simulink model "quatercar_suspension"  (R2022b)
settings: Solver=VariableStepAuto  StartTime=0.0  StopTime=10.0  RelTol=1e-3
undefined symbols (not defined in the file or in its folder): c, k, m
settings Model: Creator=admin  LastModifiedBy=admin
settings SolverCC: AlgebraicLoopSolver=TrustRegion
settings DebuggingCC: UnconnectedInputMsg=warning  UnconnectedOutputMsg=warning  UnconnectedLineMsg=warning  SFMachineParentedDataDiag=warning
settings ModelReferenceCC: EnableRefExpFcnMdlSchedulingChecks=on
settings RTWCC: DLArmComputeVersion=19.05

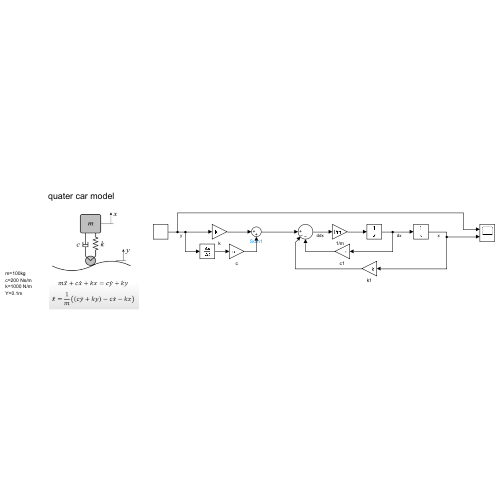
[thumbnail: Simulink's stored preview of the top-level diagram]
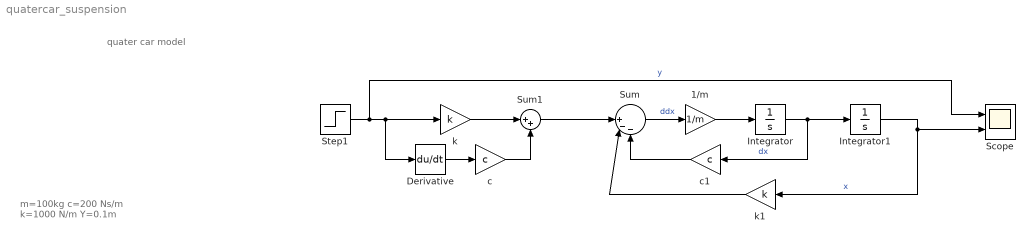
== system quatercar_suspension ==
  note: m=100kg
      | c=200 Ns/m
      | k=1000 N/m
      | Y=0.1m
  note: quater car model
  1/m : Gain  Gain=1/m
  Derivative : Derivative
  Integrator : Integrator
  Integrator1 : Integrator
  Scope : Scope  NumInputPorts=2
  Step1 : Step  After=0.1  SampleTime=0
  Sum : Sum  Inputs=||+--
  Sum1 : Sum  Inputs=|++
  c : Gain  Gain=c
  c1 : Gain  Gain=c
  k : Gain  Gain=k
  k1 : Gain  Gain=k
  wires:
  Step1/1 -> Scope/1, k/1, Derivative/1  "y"
  k/1 -> Sum1/1
  Derivative/1 -> c/1
  c/1 -> Sum1/2
  k1/1 -> Sum/2
  Sum1/1 -> Sum/1
  c1/1 -> Sum/3
  Sum/1 -> 1/m/1  "ddx"
  1/m/1 -> Integrator/1
  Integrator/1 -> c1/1, Integrator1/1  "dx"
  Integrator1/1 -> Scope/2, k1/1  "x"
